simulink model "single_robot"  (R2014a)
settings: Solver=ode15s  StartTime=0.0  StopTime=20  RelTol=1e-3
undefined symbols (not defined in the file): ASM0001, RootGround, RootPart
libraries: mblibv1 x11, fuzblock x3, simulink x1
settings Model: Creator=mohammad tariq  LastModifiedBy=lolo
settings SolverCC: ZeroCrossAlgorithm=Adaptive
settings DebuggingCC: UnderspecifiedInitializationDetection=Classic  StateNameClashWarn=warning
settings SimMechanicsCC: VisDuringSimulation=on

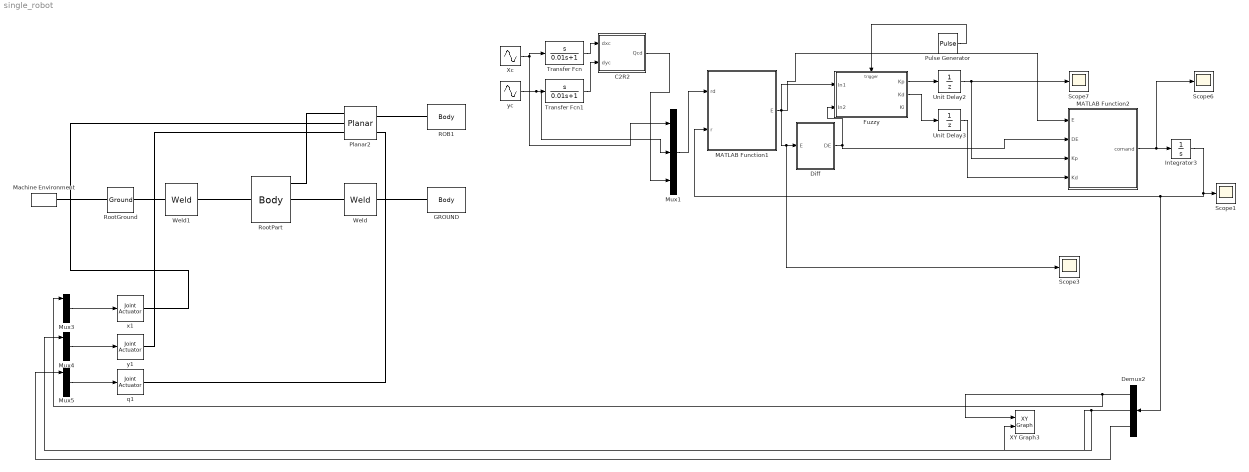
== system single_robot ==
  C2R2 : MATLAB Function  TreatAsAtomicUnit=on
  Demux2 : Demux  Outputs=3
  Diff : Subsystem
  Fuzzy : Subsystem
  GROUND : mblibv1/Bodies/Body  LConnTagsString=CS2  UpdateFromCAD=on  PMImportedID=39  DialogClass=MechanicalBodyBlock  Mass=39.3701  MassUnits=kg  InertiaUnits=kg*m^2  Inertia=[0.000328084,0,0;0,0.000328084,0;0,0,0.000656168]  Shape=Cylinder  ShapeDims=[1 1]  ShapeUnits=m  ShapeUse=false  Density=1  DensityUnits=kg/m^3  DensityUse=false  GraphicsMode=GFXFILE  GraphicsFileName=GROUND_prt.stl  BodyColorSelMode=COLORPALETTE  BodyColor=[1;1;0]  AttachedToCS=CS1  CG=Right$CG$[0 0 0.005]$WORLD$WORLD$mm$[1 0 0;0 1 0;0 0 1]$3x3 Transform$rad$WORLD$false$39::CG(AUTOGEN)  WorkingFrames=Right$CS1$[0 0 0]$WORLD$WORLD$mm$[1 0 0;0 1 0;0 0 1]$3x3 Transform$rad$WORLD$false$39::CS1(AUTOGEN)#Left$CS2$[-0.00200803 0 0.00662651]$WORLD$WORLD$mm$[1 0 0;0 1 0;0 0 1]$3x3 Transform$rad$WORLD$true$:-:39::39(AUTOGEN)  CGPos=[0 0 0.005]  CGRot=[1 0 0;0 1 0;0 0 1]  CS0Pos=[]  CS0Rot=[]  CS1Pos=[0 0 0]  CS1Rot=[1 0 0;0 1 0;0 0 1]  CS2Pos=[-0.00200803 0 0.00662651]  CS2Rot=[1 0 0;0 1 0;0 0 1]  CS3Pos=[]  CS3Rot=[]  CS4Pos=[]  CS4Rot=[]  CS5Pos=[]  CS5Rot=[]  CS6Pos=[]  CS6Rot=[]  CS7Pos=[]  CS7Rot=[]  CS8Pos=[]  CS8Rot=[]  CS9Pos=[]  CS9Rot=[]  CS10Pos=[]  CS10Rot=[]  CS11Pos=[]  CS11Rot=[]  CS12Pos=[]  CS12Rot=[]  CS13Pos=[]  CS13Rot=[]  CS14Pos=[]  CS14Rot=[]  CS15Pos=[]  CS15Rot=[]  CS16Pos=[]  CS16Rot=[]  CS17Pos=[]  CS17Rot=[]  CS18Pos=[]  CS18Rot=[]  CS19Pos=[]  CS19Rot=[]  CS20Pos=[]  CS20Rot=[]
  Integrator3 : Integrator  InitialCondition=[0 1 0 ]
  MATLAB Function1 : MATLAB Function  TreatAsAtomicUnit=on
  MATLAB Function2 : MATLAB Function  TreatAsAtomicUnit=on
  Machine Environment : mblibv1/Bodies/Machine Environment  PortType=env  PhysicalDomain=Mechanical  DialogTemplateClass=MECH.MachineEnvironment  SyncWhenCopied=off  Gravity=[0 0 0]  GravityUnits=m/s^2  GravityAsSignal=off  Dimensionality=Auto-detect  AnalysisType=Forward dynamics  LinearAssemblyTolerance=1e-3  LinearAssemblyToleranceUnits=m  AngularAssemblyTolerance=1e-3  AngularAssemblyToleranceUnits=rad  ConstraintSolverType=Stabilizing  ConstraintRelTolerance=1e-4  ConstraintAbsTolerance=1e-4  UseRobustSingularityHandling=off  RedundancyAnalysisToleranceType=Automatically select tolerance  RedundancyAnalysisTolerance=1e-14  StatePerturbationType=Fixed  PerturbationSize=1e-5  VisualizeMachine=on  BodyVisualizationType=Use model default body geometries  BodyColorSelMode=Use model default  DefaultBodyColor=[1 0 0]
  Mux{1,3..5} (4 alike) : Mux  Inputs=3
  Planar2 : mblibv1/Joints/Planar  LConnTagsString=__newl0|SA1|SA2  RConnTagsString=__newr0|SA1  UpdateFromCAD=on  NumSAPorts=3  CutJoint=off  MarkAsCut=off  Primitives=prismatic_prismatic  PrimitiveProps=P1$World$[1,0,0]$prismatic#P2$World$[0,1,0]$prismatic#R1$World$[0,0,1]$revolute  DialogClass=JointBlock  P1Axis=[1,0,0]  P2Axis=[0,1,0]  R1Axis=[0,0,1]
  Pulse Generator : DiscretePulseGenerator  PulseType=Time based  Period=0.5  PulseWidth=5
  ROB1 : mblibv1/Bodies/Body  LConnTagsString=CS2  UpdateFromCAD=on  PMImportedID=40  DialogClass=MechanicalBodyBlock  Mass=0.738189  MassUnits=kg  InertiaUnits=kg*m^2  Inertia=[1.34309e-08,0,0;0,1.11526e-08,0;0,0,2.33532e-08]  Shape=Cylinder  ShapeDims=[1 1]  ShapeUnits=m  ShapeUse=false  Density=1  DensityUnits=kg/m^3  DensityUse=false  GraphicsMode=GFXFILE  GraphicsFileName=ROB1_prt.stl  BodyColorSelMode=COLORPALETTE  BodyColor=[0 1 0]  AttachedToCS=CS1  CG=Right$CG$[-0.0555556 0 0.05]$WORLD$WORLD$mm$[1 0 0;0 1 0;0 0 1]$3x3 Transform$rad$WORLD$false$40::CG(AUTOGEN)  WorkingFrames=Right$CS1$[0 0 0]$WORLD$WORLD$mm$[1 0 0;0 1 0;0 0 1]$3x3 Transform$rad$WORLD$false$40::CS1(AUTOGEN)#Left$CS2$[0 0 0]$WORLD$WORLD$mm$[1 0 0;0 1 0;0 0 1]$3x3 Transform$rad$WORLD$true$:-:ASM0001/RootPart::40(AUTOGEN)  CGPos=[-0.0555556 0 0.05]  CGRot=[1 0 0;0 1 0;0 0 1]  CS0Pos=[]  CS0Rot=[]  CS1Pos=[0 0 0]  CS1Rot=[1 0 0;0 1 0;0 0 1]  CS2Pos=[0 0 0]  CS2Rot=[1 0 0;0 1 0;0 0 1]  CS3Pos=[]  CS3Rot=[]  CS4Pos=[]  CS4Rot=[]  CS5Pos=[]  CS5Rot=[]  CS6Pos=[]  CS6Rot=[]  CS7Pos=[]  CS7Rot=[]  CS8Pos=[]  CS8Rot=[]  CS9Pos=[]  CS9Rot=[]  CS10Pos=[]  CS10Rot=[]  CS11Pos=[]  CS11Rot=[]  CS12Pos=[]  CS12Rot=[]  CS13Pos=[]  CS13Rot=[]  CS14Pos=[]  CS14Rot=[]  CS15Pos=[]  CS15Rot=[]  CS16Pos=[]  CS16Rot=[]  CS17Pos=[]  CS17Rot=[]  CS18Pos=[]  CS18Rot=[]  CS19Pos=[]  CS19Rot=[]  CS20Pos=[]  CS20Rot=[]
  RootGround : mblibv1/Bodies/Ground  UpdateFromCAD=on  PMImportedID=RootGround  LeftPortType=env  RightPortType=workingframe  PhysicalDomain=Mechanical  DialogClass=GroundBlock  CoordPosition=[-0.00200803,0,0.00662651]  CoordPositionUnits=mm  StateVectorMgrId=2  MachineId=[3 0]  ShowEnvPort=on  ParameterChecksum=[3235804778, 1106055459, 4068079292, 123382310]  TopologyChecksum=[1072569561, 1126036512, 910051422, 1001480646]
  RootPart : mblibv1/Bodies/Body  LConnTagsString=CS5  RConnTagsString=CS2|CS3|CS4  UpdateFromCAD=on  PMImportedID=ASM0001/RootPart  DialogClass=MechanicalBodyBlock  Mass=0  MassUnits=kg  InertiaUnits=kg*m^2  Inertia=[0,0,0;0,0,0;0,0,0]  Shape=Cylinder  ShapeDims=[1 1]  ShapeUnits=m  ShapeUse=false  Density=1  DensityUnits=kg/m^3  DensityUse=false  GraphicsMode=MACHINE_DEFAULT  BodyColorSelMode=MACHINE_DEFAULT  BodyColor=[1;0;0]  AttachedToCS=CS1  CG=Right$CG$[-0.00200803 0 0.00662651]$WORLD$WORLD$mm$[1 0 0;0 1 0;0 0 1]$3x3 Transform$rad$WORLD$false$ASM0001/RootPart::CG(AUTOGEN)  WorkingFrames=Right$CS1$[0 0 0]$WORLD$WORLD$mm$[1 0 0;0 1 0;0 0 1]$3x3 Transform$rad$WORLD$false$ASM0001/RootPart::CS1(AUTOGEN)#Right$CS2$[0 0 0]$WORLD$WORLD$mm$[1 0 0;0 1 0;0 0 1]$3x3 Transform$rad$WORLD$true$:-:ASM0001/RootPart::ASM0001/RootPart(AUTOGEN)#Right$CS3$[-0.00200803 0 0.00662651]$WORLD$WORLD$mm$[1 0 0;0 1 0;0 0 1]$3x3 Transform$rad$WORLD$true$:-:39::ASM0001/RootPart(AUTOGEN)#Right$CS4$[0 0 0]$WORLD$WORLD$mm$[1 0 0;0 1 0;0 0 1]$3x3 Transform$rad$WORLD$true$:-:ASM0001/RootPart::ASM0001/RootPart(AUTOGEN)#Left$CS5$[-0.00200803 0 0.00662651]$WORLD$WORLD$mm$[1 0 0;0 1 0;0 0 1]$3x3 Transform$rad$WORLD$true$ASM0001/RootPart:-:RootGround::ASM0001/RootPart(AUTOGEN)  CGPos=[-0.00200803 0 0.00662651]  CGRot=[1 0 0;0 1 0;0 0 1]  CS0Pos=[]  CS0Rot=[]  CS1Pos=[0 0 0]  CS1Rot=[1 0 0;0 1 0;0 0 1]  CS2Pos=[0 0 0]  CS2Rot=[1 0 0;0 1 0;0 0 1]  CS3Pos=[-0.00200803 0 0.00662651]  CS3Rot=[1 0 0;0 1 0;0 0 1]  CS4Pos=[0 0 0]  CS4Rot=[1 0 0;0 1 0;0 0 1]  CS5Pos=[-0.00200803 0 0.00662651]  CS5Rot=[1 0 0;0 1 0;0 0 1]  CS6Pos=[]  CS6Rot=[]  CS7Pos=[]  CS7Rot=[]  CS8Pos=[]  CS8Rot=[]  CS9Pos=[]  CS9Rot=[]  CS10Pos=[]  CS10Rot=[]  CS11Pos=[]  CS11Rot=[]  CS12Pos=[]  CS12Rot=[]  CS13Pos=[]  CS13Rot=[]  CS14Pos=[]  CS14Rot=[]  CS15Pos=[]  CS15Rot=[]  CS16Pos=[]  CS16Rot=[]  CS17Pos=[]  CS17Rot=[]  CS18Pos=[]  CS18Rot=[]  CS19Pos=[]  CS19Rot=[]  CS20Pos=[]  CS20Rot=[]
  Scope{1,3,6..7} (4 alike) : Scope
      Scope1 settings: YMin=-3
      Scope3 settings: YMin=-1  YMax=6.5
      Scope6 settings: YMax=32.5  SaveName=ScopeData5
      Scope7 settings: YMin=-0.35  YMax=0.35  SaveName=ScopeData6
  Transfer Fcn : TransferFcn  Numerator=[1 0]  Denominator=[0.01 1]
  Transfer Fcn1 : TransferFcn  Numerator=[1 0]  Denominator=[0.01 1]
  Unit Delay2 : UnitDelay  InitialCondition=[0 0 0]  SampleTime=0.5
  Unit Delay3 : UnitDelay  InitialCondition=[0 0 0]  SampleTime=0.5
  Weld : mblibv1/Joints/Weld  LConnTagsString=__newl0  RConnTagsString=__newr0  UpdateFromCAD=on  PMImportedID=:-:39  NumSAPorts=0  CutJoint=off  MarkAsCut=off  Primitives=weld  PrimitiveProps=W$WORLD$[0.57735,0.57735,0.57735]$weld  DialogClass=JointBlock  WAxis=[0.57735,0.57735,0.57735]
  Weld1 : mblibv1/Joints/Weld  LConnTagsString=__newl0  RConnTagsString=__newr0  UpdateFromCAD=on  PMImportedID=ASM0001/RootPart:-:RootGround  NumSAPorts=0  CutJoint=off  MarkAsCut=off  Primitives=weld  PrimitiveProps=W$WORLD$[0.57735,0.57735,0.57735]$weld  DialogClass=JointBlock  WAxis=[0.57735,0.57735,0.57735]
  XY Graph3 : simulink/Sinks/XY Graph  xmin=-10  xmax=10  ymin=-10  ymax=10  st=-1
  Xc : Sin  Amplitude=5  SampleTime=0
  q1 : mblibv1/Sensors &  Actuators/Joint Actuator  UpdateFromCAD=off  PhysicalDomain=Mechanical  PortType=blob  ActuationStyle=Motion  AngleUnits=rad  ArcVelocityUnits=deg/s  ArcAccelerationUnits=deg/s^2  CoordPositionUnits=mm  VelocityUnits=m/s  AccelerationUnits=m/s^2  ForceUnits=N  TorqueUnits=N*m  ActiveIO=on  Width=3  DialogClass=MechanicalActuatorBlock  Primitive=R1  ReferenceFrame=Absolute (World)
  x1 : mblibv1/Sensors &  Actuators/Joint Actuator  UpdateFromCAD=off  PhysicalDomain=Mechanical  PortType=blob  ActuationStyle=Motion  AngleUnits=deg  ArcVelocityUnits=deg/s  ArcAccelerationUnits=deg/s^2  CoordPositionUnits=mm  VelocityUnits=m/s  AccelerationUnits=m/s^2  ForceUnits=N  TorqueUnits=N*m  ActiveIO=on  Width=3  DialogClass=MechanicalActuatorBlock  Primitive=P1  ReferenceFrame=Absolute (World)
  y1 : mblibv1/Sensors &  Actuators/Joint Actuator  UpdateFromCAD=off  PhysicalDomain=Mechanical  PortType=blob  ActuationStyle=Motion  AngleUnits=deg  ArcVelocityUnits=deg/s  ArcAccelerationUnits=deg/s^2  CoordPositionUnits=mm  VelocityUnits=m/s  AccelerationUnits=m/s^2  ForceUnits=N  TorqueUnits=N*m  ActiveIO=on  Width=3  DialogClass=MechanicalActuatorBlock  Primitive=P2  ReferenceFrame=Absolute (World)
  yc : Sin  Amplitude=5  Phase=pi/2  SampleTime=0
  wires:
  Mux3/1 -> x1/1
  Mux4/1 -> y1/1
  Mux5/1 -> q1/1
  Xc/1 -> Mux1/1, Transfer Fcn/1
  yc/1 -> Transfer Fcn1/1, Mux1/2
  Transfer Fcn/1 -> C2R2/1(dxc)
  Transfer Fcn1/1 -> C2R2/2(dyc)
  C2R2/1(Qcd) -> Mux1/3
  Mux1/1 -> MATLAB Function1/1(rd)
  MATLAB Function1/1(E) -> Scope3/1, Diff/1(E), Fuzzy/1(In1), MATLAB Function2/1(E)
  Unit Delay2/1 -> MATLAB Function2/3(Kp), Scope7/1
  Unit Delay3/1 -> MATLAB Function2/4(Kd)
  MATLAB Function2/1(comand) -> Scope6/1, Integrator3/1
  Diff/1(DE) -> Fuzzy/2(In2), MATLAB Function2/2(DE)
  Fuzzy/1(Kp) -> Unit Delay2/1
  Fuzzy/2(Kd) -> Unit Delay3/1
  Pulse Generator/1 -> Fuzzy/Trigger
  Demux2/1 -> Mux3/1, XY Graph3/1
  Demux2/2 -> Mux4/1, XY Graph3/2
  Integrator3/1 -> Scope1/1, Demux2/1, MATLAB Function1/2(r)
  Demux2/3 -> Mux5/1
  connections:
  Planar2/LConn1 -- RootPart/RConn1
  Planar2/RConn1 -- ROB1/LConn1
  RootPart/RConn2 -- Weld/LConn1
  Weld/RConn1 -- GROUND/LConn1
  RootGround/RConn1 -- Weld1/LConn1
  Weld1/RConn1 -- RootPart/LConn1
  RootGround/LConn1 -- Machine Environment/RConn1
  x1/RConn1 -- Planar2/LConn2
  q1/RConn1 -- Planar2/RConn2
  y1/RConn1 -- Planar2/LConn3

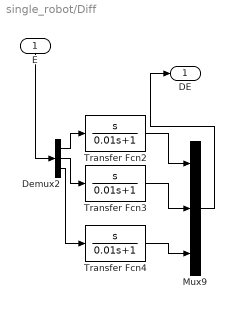
== system single_robot/Diff ==
  E : Inport
  Demux2 : Demux  Outputs=3
  Mux9 : Mux  Inputs=3
  Transfer Fcn2 : TransferFcn  Numerator=[1 0]  Denominator=[0.01 1]
  Transfer Fcn3 : TransferFcn  Numerator=[1 0]  Denominator=[0.01 1]
  Transfer Fcn4 : TransferFcn  Numerator=[1 0]  Denominator=[0.01 1]
  DE : Outport
  wires:
  Transfer Fcn4/1 -> Mux9/3
  Demux2/2 -> Transfer Fcn3/1
  Transfer Fcn3/1 -> Mux9/2
  Transfer Fcn2/1 -> Mux9/1
  Demux2/1 -> Transfer Fcn2/1
  Demux2/3 -> Transfer Fcn4/1
  Mux9/1 -> DE/1
  E/1 -> Demux2/1

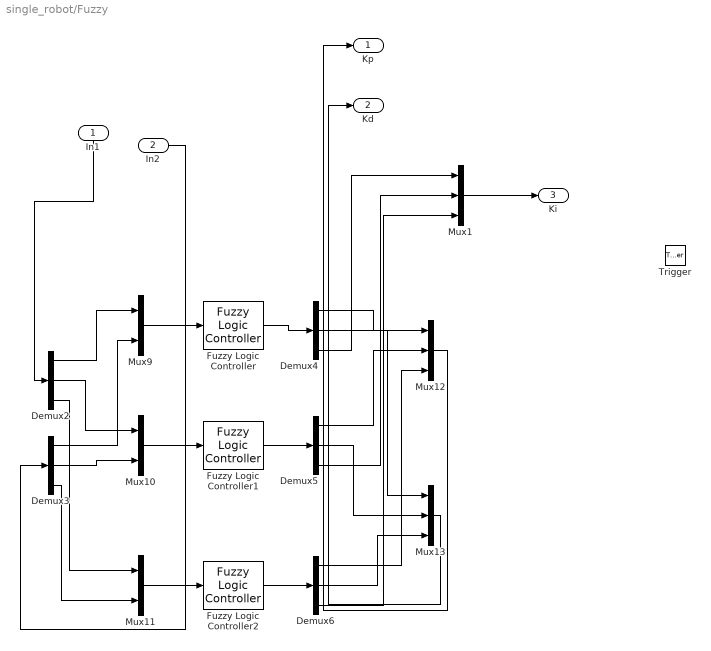
== system single_robot/Fuzzy ==
  In1 : Inport
  In2 : Inport  Port=2
  Trigger : TriggerPort  PortDimensions=1
  Demux{2..6} (5 alike) : Demux  Outputs=3
  Fuzzy Logic Controller : fuzblock/Fuzzy Logic  Controller  fis=readfis('C1.fis')
  Fuzzy Logic Controller1 : fuzblock/Fuzzy Logic  Controller  fis=readfis('C1.fis')
  Fuzzy Logic Controller2 : fuzblock/Fuzzy Logic  Controller  fis=readfis('C1.fis')
  Mux1 : Mux  Inputs=3
  Mux10 : Mux  Inputs=2
  Mux11 : Mux  Inputs=2
  Mux12 : Mux  Inputs=3
  Mux13 : Mux  Inputs=3
  Mux9 : Mux  Inputs=2
  Kp : Outport
  Kd : Outport  Port=2
  Ki : Outport  Port=3
  wires:
  Mux11/1 -> Fuzzy Logic Controller2/1
  Demux3/1 -> Mux9/2
  Demux3/3 -> Mux11/2
  Demux2/2 -> Mux10/1
  Demux2/1 -> Mux9/1
  Demux2/3 -> Mux11/1
  Mux13/1 -> Kd/1
  Mux12/1 -> Kp/1
  Demux4/2 -> Mux13/1
  Demux5/2 -> Mux13/2
  Demux6/1 -> Mux12/3
  Mux9/1 -> Fuzzy Logic Controller/1
  Demux5/1 -> Mux12/2
  Mux10/1 -> Fuzzy Logic Controller1/1
  Demux6/2 -> Mux13/3
  Fuzzy Logic Controller1/1 -> Demux5/1
  Fuzzy Logic Controller2/1 -> Demux6/1
  Fuzzy Logic Controller/1 -> Demux4/1
  In2/1 -> Demux3/1
  Demux4/1 -> Mux12/1
  In1/1 -> Demux2/1
  Demux3/2 -> Mux10/2
  Mux1/1 -> Ki/1
  Demux4/3 -> Mux1/1
  Demux5/3 -> Mux1/2
  Demux6/3 -> Mux1/3

== matlab function single_robot/C2R2 ==
  data: dxc input; dyc input; Qcd output
function Qcd    = fcn(dxc,dyc)

Qcd = atan2(dyc,dxc);

% dq1 = (dy1/x1-(y1*dx1)/x1^2)*(tan(y1/x1)^2+1);

== matlab function single_robot/MATLAB Function2 ==
  data: E input; DE input; Kp input; Kd input; comand output
function comand  = fcn(E,DE,Kp,Kd)
comand=zeros(3,1);
comand(1)=E(1)*(Kp(1)+5)+DE(1)*(0.5*Kd(1)+0.5);
comand(2)=E(2)*(Kp(2)+5)+DE(2)*(0.5*Kd(2)+0.5);
comand(3)=E(3)*(Kp(3)+5)+DE(3)*(0.5*Kd(3)+0.5);

== matlab function single_robot/MATLAB Function1 ==
  data: rd input; E output; r input
function E = fcn(rd,r)
E=zeros(3,1);
% r(3)=atan2(sin(r(3)),cos(r(3)));

E=rd-r;
 E(3)=atan2(sin(E(3)),cos(E(3)));
